simulink model "ysw3_47"  (R2014a)
settings: Solver=ode45  StartTime=0.0  StopTime=10.0  RelTol=1e-3
settings Model: Creator=Administrator  LastModifiedBy=Administrator

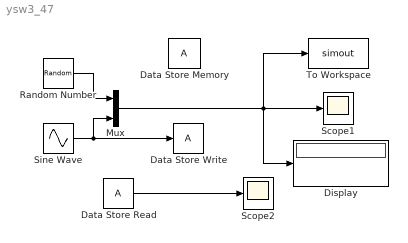
== system ysw3_47 ==
  Data Store Memory : DataStoreMemory  ReadBeforeWriteMsg=warning  WriteAfterWriteMsg=warning  WriteAfterReadMsg=warning  InitialValue=25  OutDataTypeStr=double
  Data Store Read : DataStoreRead
  Data Store Write : DataStoreWrite
  Display : Display
  Mux : Mux  Inputs=2
  Random Number : RandomNumber  SampleTime=0.1
  Scope1 : Scope
      settings: TimeRange=10
  Scope2 : Scope
      settings: TimeRange=10
  Sine Wave : Sin  SampleTime=0.1
  To Workspace : ToWorkspace  VariableName=simout  SaveFormat=Timeseries  SampleTime=-1
  wires:
  Random Number/1 -> Mux/1
  Sine Wave/1 -> Data Store Write/1, Mux/2
  Mux/1 -> To Workspace/1, Scope1/1, Display/1
  Data Store Read/1 -> Scope2/1
